simulink model "tut3"  (R2012b)
settings: Solver=ode45  StartTime=0.0  StopTime=8192  RelTol=1e-3
undefined symbols (not defined in the file): gcbh, pfb_coeff_gen_calc, xlBlockLoadCallback
libraries: xbsIndex_r4 x2165, casper_library_misc x93, casper_library_delays x38, xps_library x10, xbsReplacements_r4 x2, casper_library_pfbs x2, simulink x1, casper_library_ffts_twiddle x1, casper_library_reorder x1
(part 21 of 31)

== system tut3/fft_wideband_real/fft_direct/butterfly2_1/twiddle_general_4mult/coeff_gen ==
  rst : Inport
  Counter : xbsIndex_r4/Counter  cnt_type=Free Running  cnt_to=Inf  operation=Up  start_count=0  cnt_by_val=1  arith_type=Unsigned  n_bits=10  bin_pt=0  load_pin=off  rst=on  en=off  explicit_period=on  period=1  dbl_ovrd=off  use_behavioral_HDL=off  implementation=Fabric  block_type=counter
  ROM : xbsIndex_r4/ROM  depth=1024  initVector="[0                    -0.0015411376953125                    -0.0030670166015625                     -0.004608154296875                     -0.006134033203125                    -0.0076751708984375                    -0.0092010498046875                          -0.0107421875                      -0.01226806640625                    -0.0138092041015625                    -0.0153350830078125                     -0.016876220703125                     -0.018402099609375                    -0.0199432373046875                    -0.0214691162109375                      -0.02301025390625                       -0.0245361328125                    -0.0260772705078125                    -0.0276031494140625                     -0.029144287109375                     -0.030670166015625                    -0.0322113037109375                    -0.0337371826171875                       -0.0352783203125                      -0.03680419921875                    -0.0383453369140625                    -0.0398712158203125                     -0.041412353515625                     -0.042938232421875                     -0.044464111328125                    -0.0460052490234375                    -0.0475311279296875                        -0.049072265625                      -0.05059814453125                    -0.0521392822265625                    -0.0536651611328125                    -0.0551910400390625                     -0.056732177734375                     -0.058258056640625                     -0.059783935546875                    -0.0613250732421875                    -0.0628509521484375                    -0.0643768310546875                         -0.06591796875                      -0.06744384765625                       -0.0689697265625                    -0.0705108642578125                    -0.0720367431640625                    -0.0735626220703125                    -0.0750885009765625                     -0.076629638671875                     -0.078155517578125                     -0.079681396484375                     -0.081207275390625                     -0.082733154296875                    -0.0842742919921875                    -0.0858001708984375                    -0.0873260498046875                    -0.0888519287109375                    -0.0903778076171875                    -0.0919036865234375                    -0.0934295654296875                        -0.094970703125                      -0.09649658203125                       -0.0980224609375                      -0.09954833984375                         -0.10107421875                      -0.10260009765625                       -0.1041259765625                      -0.10565185546875                        -0.107177734375                      -0.10870361328125                       -0.1102294921875                    -0.1117401123046875                    -0.1132659912109375                    -0.1147918701171875                    -0.1163177490234375                    -0.1178436279296875                    -0.1193695068359375                    -0.1208953857421875                     -0.122406005859375                     -0.123931884765625                     -0.125457763671875                     -0.126983642578125                    -0.1284942626953125                    -0.1300201416015625                    -0.1315460205078125                        -0.133056640625                      -0.13458251953125                    -0.1360931396484375                    -0.1376190185546875                    -0.1391448974609375                     -0.140655517578125                     -0.142181396484375                    -0.1436920166015625                    -0.1452178955078125                        -0.146728515625                      -0.14825439453125                    -0.1497650146484375                     -0.151275634765625                     -0.152801513671875                    -0.1543121337890625                      -0.15582275390625 ...(+35900 chars)]"  distributed_mem=Block RAM  rst=off  init_reg=0  en=off  latency=2  gui_display_data_type=Fixed-point  arith_type="Signed  (2's comp)"  n_bits=18  bin_pt=16  preci_type=Single  exp_width=8  frac_width=24  dbl_ovrd=off  optimize=Area  use_rpm=on  block_type=sprom
  ROM1 : xbsIndex_r4/ROM  depth=1024  initVector="[-1                                     -1                                     -1                    -0.9999847412109375                    -0.9999847412109375                     -0.999969482421875                    -0.9999542236328125                      -0.99993896484375                    -0.9999237060546875                     -0.999908447265625                       -0.9998779296875                    -0.9998626708984375                    -0.9998321533203125                    -0.9998016357421875                    -0.9997711181640625                    -0.9997406005859375                      -0.99969482421875                     -0.999664306640625                    -0.9996185302734375                      -0.99957275390625                    -0.9995269775390625                     -0.999481201171875                    -0.9994354248046875                    -0.9993743896484375                      -0.99932861328125                        -0.999267578125                      -0.99920654296875                       -0.9991455078125                      -0.99908447265625                    -0.9990081787109375                    -0.9989471435546875                     -0.998870849609375                    -0.9987945556640625                      -0.99871826171875                    -0.9986419677734375                     -0.998565673828125                      -0.99847412109375                     -0.998382568359375                    -0.9983062744140625                    -0.9982147216796875                    -0.9981231689453125                     -0.998016357421875                       -0.9979248046875                    -0.9978179931640625                    -0.9977264404296875                      -0.99761962890625                    -0.9975128173828125                     -0.997406005859375                     -0.997283935546875                    -0.9971771240234375                    -0.9970550537109375                       -0.9969482421875                        -0.996826171875                       -0.9967041015625                    -0.9965667724609375                    -0.9964447021484375                     -0.996307373046875                     -0.996185302734375                    -0.9960479736328125                      -0.99591064453125                    -0.9957733154296875                    -0.9956207275390625                       -0.9954833984375                     -0.995330810546875                      -0.99517822265625                     -0.995025634765625                        -0.994873046875                     -0.994720458984375                      -0.99456787109375                    -0.9944000244140625                    -0.9942474365234375                      -0.99407958984375                    -0.9939117431640625                     -0.993743896484375                     -0.993560791015625                    -0.9933929443359375                    -0.9932098388671875                    -0.9930267333984375                    -0.9928436279296875                    -0.9926605224609375                    -0.9924774169921875                    -0.9922943115234375                     -0.992095947265625                     -0.991912841796875                    -0.9917144775390625                      -0.99151611328125                    -0.9913177490234375                    -0.9911041259765625                      -0.99090576171875                     -0.990692138671875                        -0.990478515625                    -0.9902801513671875                      -0.99005126953125                     -0.989837646484375                       -0.9896240234375                    -0.9893951416015625                    -0.9891815185546875                      -0.98895263671875                    -0.9887237548828125                     -0.988494873046875                     -0.988250732421875                    -0.9880218505859375                    -0.9877777099609375 ...(+35901 chars)]"  distributed_mem=Block RAM  rst=off  init_reg=0  en=off  latency=2  gui_display_data_type=Fixed-point  arith_type="Signed  (2's comp)"  n_bits=18  bin_pt=16  preci_type=Single  exp_width=8  frac_width=24  dbl_ovrd=off  optimize=Area  use_rpm=on  block_type=sprom
  Slice : xbsIndex_r4/Slice  nbits=10  boolean_output=off  mode=Upper Bit Location + Width  bit1=0  base1=MSB of Input  bit0=0  base0=LSB of Input  dbl_ovrd=off  block_type=slice
  ri_to_c : casper_library_misc/ri_to_c
  w : Outport
  wires:
  ri_to_c/1 -> w/1
  rst/1 -> Counter/1
  Counter/1 -> Slice/1
  Slice/1 -> ROM/1, ROM1/1
  ROM/1 -> ri_to_c/1
  ROM1/1 -> ri_to_c/2
